simulink model "SwingSimulation"  (Simulink 9.3)
settings: Solver=ode4  StartTime=0.0  StopTime=10  FixedStep=0.001  RelTol=1e-3
values from neighbouring files (symbols this model uses):
  G_SI = 9.81    [dfile_o.m]
  J_SI = 0.5 * M_SI * R1_SI * R1_SI    (= 0.0047357219357)    [dfile_o.m]
  L2_SI = L2 * 0.0254    (= 0.7874)    [dfile_o.m]
libraries: simulink x7
settings Model: Creator=jwagner  LastModifiedBy=ameya
settings DataIOCC: SaveFormat=Dataset  SignalLoggingSaveFormat=Dataset
settings OptimizationCC: LifeSpan=auto
settings DebuggingCC: UnderspecifiedInitializationDetection=Simplified  MergeDetectMultiDrivingBlocksExec=error  FcnCallInpInsideContextMsg=error  PregeneratedLibrarySubsystemCodeDiagnostic=none  SFUnexpectedBacktrackingDiag=error  SFNoUnconditionalDefaultTransitionDiag=error  SFExecutionAtInitializationDiag=warning
settings HardwareCC: ProdBitPerPointer=64  ProdBitPerSizeT=64  ProdBitPerPtrDiffT=64  ProdLargestAtomicFloat=Float  ProdIntDivRoundTo=Zero  ProdEndianess=LittleEndian  ProdWordSize=64  ProdHWDeviceType=Intel->x86-64 (Windows64)
settings ModelReferenceCC: PropagateSignalLabelsOutOfModel=on
settings GRTTargetCC: TargetLangStandard=C99 (ISO)  CombineOutputUpdateFcns=on  GRTInterface=off
settings ConfigComp: CovMetricSettings=dwe  CovHtmlReporting=off  CovSaveCumulativeToWorkspaceVar=off  CovSaveSingleToWorkspaceVar=off  CovExternalEMLEnable=on

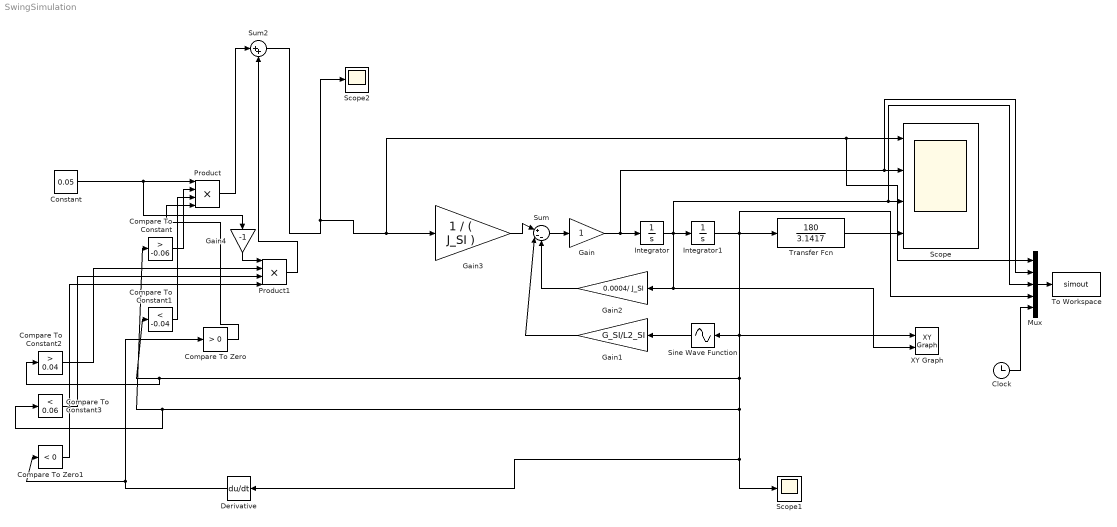
== system SwingSimulation ==
  Clock : Clock
  Compare To Constant : simulink/Logic and Bit Operations/Compare To Constant  relop=>  const=-0.06  OutDataTypeStr=boolean
  Compare To Constant1 : simulink/Logic and Bit Operations/Compare To Constant  relop=<  const=-0.04  OutDataTypeStr=boolean
  Compare To Constant2 : simulink/Logic and Bit Operations/Compare To Constant  relop=>  const=0.04  OutDataTypeStr=boolean
  Compare To Constant3 : simulink/Logic and Bit Operations/Compare To Constant  relop=<  const=0.06  OutDataTypeStr=boolean
  Compare To Zero : simulink/Logic and Bit Operations/Compare To Zero  relop=>  OutDataTypeStr=boolean
  Compare To Zero1 : simulink/Logic and Bit Operations/Compare To Zero  relop=<  OutDataTypeStr=boolean
  Constant : Constant  Value=0.05
  Derivative : Derivative
  Gain : Gain
  Gain1 : Gain  Gain=G_SI/L2_SI
  Gain2 : Gain  Gain=0.0004/ J_SI
  Gain3 : Gain  Gain=1 / ( J_SI )
  Gain4 : Gain  Gain=-1
  Integrator : Integrator
  Integrator1 : Integrator  InitialCondition=0.05
  Mux : Mux  Inputs=5
  Product : Product  Inputs=4
  Product1 : Product  Inputs=4
  Scope : Scope  NumInputPorts=4
  Scope1 : Scope
  Scope2 : Scope
  Sine Wave Function : Sin  TimeSource=Use external signal  SampleTime=0
  Sum : Sum  Inputs=|+--
  Sum2 : Sum  Inputs=|++
  To Workspace : ToWorkspace  VariableName=simout  SampleTime=-1
      settings: Save2DSignal=2-D array (concatenate along first dimension)
  Transfer Fcn : TransferFcn  Numerator=180  Denominator=3.1417
  XY Graph : simulink/Sinks/XY Graph  xmin=-5  xmax=5  ymin=-5  ymax=5  st=-1
  wires:
  Gain/1 -> Mux/2, Scope/2, Integrator/1
  Integrator/1 -> Mux/3, Scope/3, XY Graph/2, Gain2/1, Integrator1/1
  Sum/1 -> Gain/1
  Sine Wave Function/1 -> Gain1/1
  Integrator1/1 -> Compare To Constant2/1, Compare To Constant1/1, Compare To Constant3/1, Compare To Constant/1, Derivative/1, Scope1/1, Sine Wave Function/1, XY Graph/1, Mux/4, Transfer Fcn/1
  Gain1/1 -> Sum/2
  Transfer Fcn/1 -> Scope/4
  Sum2/1 -> Gain3/1, Mux/1, Scope/1, Scope2/1
  Gain3/1 -> Sum/1
  Gain2/1 -> Sum/3
  Mux/1 -> To Workspace/1
  Clock/1 -> Mux/5
  Constant/1 -> Gain4/1, Product/1
  Compare To Constant/1 -> Product/2
  Product/1 -> Sum2/1
  Product1/1 -> Sum2/2
  Derivative/1 -> Compare To Zero1/1, Compare To Zero/1
  Compare To Constant1/1 -> Product/3
  Compare To Zero/1 -> Product/4
  Compare To Constant2/1 -> Product1/2
  Compare To Constant3/1 -> Product1/3
  Compare To Zero1/1 -> Product1/4
  Gain4/1 -> Product1/1
